simulink model "Color_Space"  (R2013b)
settings: Solver=ode45  StartTime=0.0  StopTime=384*512  RelTol=1e-3
undefined symbols (not defined in the file or in its folder): gray
libraries: xbsIndex_r4 x29, dspsigattribs x9, visionsinks x3, visionsources x1
settings Model: Creator=Sechw  LastModifiedBy=Sechw

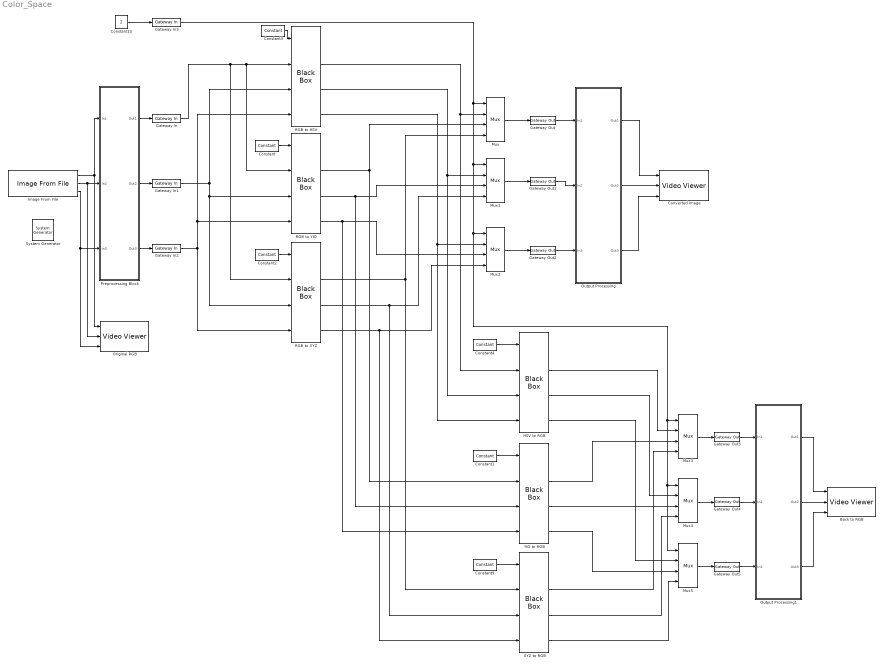
== system Color_Space ==
  " System Generator" : xbsIndex_r4/ System Generator  Tag=genX  xilinxfamily=virtex5  part=xc5vlx110t  speed=-1  package=ff1136  synthesis_tool=XST  clock_wrapper=Clock Enables  directory=./netlist  proj_type=Project Navigator  Synth_file=XST Defaults  Impl_file=ISE Defaults  testbench=off  simulink_period=1  sysclk_period=10  dcm_input_clock_period=10  incr_netlist=off  trim_vbits=Everywhere in SubSystem  dbl_ovrd=According to Block Masks  core_generation=According to Block Masks  run_coregen=off  deprecated_control=off  eval_field=0  block_type=sysgen
  Back to RGB : visionsinks/Video Viewer  inputType=Obsolete7b  imagePorts=Separate color signals  useColorMap=off  colormapValue=gray(256)  specRange=off  minInputVal=0  maxInputVal=255  FigPos=[230 612 675 424]  AxisZoom=on  trueSizedOnce=off  OpenAtMdlStart=on  DefaultConfigurationName=vipscopes.VideoViewerScopeCfg
  Constant{,1..4,9} (6 alike) : xbsIndex_r4/Constant  const=0  gui_display_data_type=Boolean  arith_type=Boolean  n_bits=16  bin_pt=14  preci_type=Single  exp_width=8  frac_width=24  explicit_period=off  period=1  equ=P=C  opselect=C  inp2=PCIN>>17  opr=+  inp1=P  carry=CIN  dbl_ovrd=off  block_type=constant
  Constant13 : Constant  Value=2
  Converted Image : visionsinks/Video Viewer  inputType=Obsolete7b  imagePorts=Separate color signals  useColorMap=off  colormapValue=gray(256)  specRange=off  minInputVal=0  maxInputVal=255  FigPos=[197 708 647 463]  AxisZoom=on  trueSizedOnce=off  OpenAtMdlStart=on  DefaultConfigurationName=vipscopes.VideoViewerScopeCfg
  Gateway In : xbsIndex_r4/Gateway In  gui_display_data_type=Fixed-point  arith_type=Unsigned  n_bits=8  bin_pt=0  preci_type=Double  exp_width=8  frac_width=24  quantization="Round  (unbiased: +/- Inf)"  overflow=Saturate  period=1  dbl_ovrd=off  timing_constraint=None  locs_specified=off  LOCs={}  UseAsADC=off  ADCChannel='1'  inherit_from_input=off  hdl_port=on  block_type=gatewayin
  Gateway In1 : xbsIndex_r4/Gateway In  gui_display_data_type=Fixed-point  arith_type=Unsigned  n_bits=8  bin_pt=0  preci_type=Double  exp_width=8  frac_width=24  quantization="Round  (unbiased: +/- Inf)"  overflow=Saturate  period=1  dbl_ovrd=off  timing_constraint=None  locs_specified=off  LOCs={}  UseAsADC=off  ADCChannel='1'  inherit_from_input=off  hdl_port=on  block_type=gatewayin
  Gateway In2 : xbsIndex_r4/Gateway In  gui_display_data_type=Fixed-point  arith_type=Unsigned  n_bits=8  bin_pt=0  preci_type=Double  exp_width=8  frac_width=24  quantization="Round  (unbiased: +/- Inf)"  overflow=Saturate  period=1  dbl_ovrd=off  timing_constraint=None  locs_specified=off  LOCs={}  UseAsADC=off  ADCChannel='1'  inherit_from_input=off  hdl_port=on  block_type=gatewayin
  Gateway In3 : xbsIndex_r4/Gateway In  gui_display_data_type=Fixed-point  arith_type=Unsigned  n_bits=2  bin_pt=0  preci_type=Single  exp_width=8  frac_width=24  quantization="Round  (unbiased: +/- Inf)"  overflow=Saturate  period=1  dbl_ovrd=off  timing_constraint=None  locs_specified=off  LOCs={}  UseAsADC=off  ADCChannel='1'  inherit_from_input=off  hdl_port=on  block_type=gatewayin
  Gateway Out{,1..5} (6 alike) : xbsIndex_r4/Gateway Out  inherit_from_input=on  hdl_port=on  timing_constraint=None  locs_specified=off  LOCs={}  UseAsDAC=off  DACChannel='1'  block_type=gatewayout
  HSV to RGB : xbsIndex_r4/Black Box  init_code=hsvtorgb_fixpt_xsgbbxcfg  sim_method=ISE Simulator  verbose=off  block_type=blackbox2
  Image From File : visionsources/Image From File  Tag=vipblks_nd  FileName=C:\Users\Sechw\Documents\MATLAB\4440\peppers.png  imagePorts=Separate color signals  Ts=inf  ImageDataType=Inherit from input image  Signed=on  WordLength=16  sdImageDataType=uint(8)  FractionLengthMode=User-defined  FractionLength=15  OutPortLabels=R|G|B
  Mux{,1..5} (6 alike) : xbsIndex_r4/Mux  inputs=3  en=off  latency=0  precision=Full  arith_type=Unsigned  n_bits=16  bin_pt=14  quantization=Truncate  overflow=Wrap  dbl_ovrd=off  block_type=mux
  Original RGB : visionsinks/Video Viewer  inputType=Obsolete7b  imagePorts=Separate color signals  useColorMap=off  colormapValue=gray(256)  specRange=off  minInputVal=0  maxInputVal=255  FigPos=[800 621 504 461]  AxisZoom=on  trueSizedOnce=off  OpenAtMdlStart=on  DefaultConfigurationName=vipscopes.VideoViewerScopeCfg
  Output Processing : Subsystem
  Output Processing1 : Subsystem
  Preprocessing Block : Subsystem
  RGB to HSV : xbsIndex_r4/Black Box  init_code=rgbtohsv_fixpt_xsgbbxcfg  sim_method=ISE Simulator  verbose=off  block_type=blackbox2
  RGB to XYZ : xbsIndex_r4/Black Box  init_code=rgbtoxyz_fixpt_xsgbbxcfg  sim_method=ISE Simulator  verbose=off  block_type=blackbox2
  RGB to YIQ : xbsIndex_r4/Black Box  init_code=rgbtoyiq_fixpt_xsgbbxcfg  sim_method=ISE Simulator  verbose=off  block_type=blackbox2
  XYZ to RGB : xbsIndex_r4/Black Box  init_code=xyztorgb_fixpt_xsgbbxcfg  sim_method=ISE Simulator  verbose=off  block_type=blackbox2
  YIQ to RGB : xbsIndex_r4/Black Box  init_code=yiqtorgb_fixpt_xsgbbxcfg  sim_method=ISE Simulator  verbose=off  block_type=blackbox2
  wires:
  Image From File/1 -> Preprocessing Block/1(In1), Original RGB/1
  Image From File/2 -> Original RGB/2, Preprocessing Block/2(In2)
  Image From File/3 -> Original RGB/3, Preprocessing Block/3(In3)
  Preprocessing Block/1(Out1) -> Gateway In/1
  Preprocessing Block/2(Out2) -> Gateway In1/1
  Preprocessing Block/3(Out3) -> Gateway In2/1
  Gateway Out/1 -> Output Processing/1(In1)
  Gateway Out1/1 -> Output Processing/2(In2)
  Gateway Out2/1 -> Output Processing/3(In3)
  Output Processing/1(Out1) -> Converted Image/1
  Output Processing/2(Out2) -> Converted Image/2
  Output Processing/3(Out3) -> Converted Image/3
  Gateway Out3/1 -> Output Processing1/1(In1)
  Gateway Out4/1 -> Output Processing1/2(In2)
  Gateway Out5/1 -> Output Processing1/3(In3)
  Output Processing1/1(Out1) -> Back to RGB/1
  Output Processing1/2(Out2) -> Back to RGB/2
  Output Processing1/3(Out3) -> Back to RGB/3
  Constant1/1 -> YIQ to RGB/1
  Constant2/1 -> RGB to XYZ/1
  Mux/1 -> Gateway Out/1
  Mux1/1 -> Gateway Out1/1
  Mux2/1 -> Gateway Out2/1
  Constant9/1 -> XYZ to RGB/1
  Mux3/1 -> Gateway Out3/1
  Mux4/1 -> Gateway Out4/1
  Mux5/1 -> Gateway Out5/1
  Constant13/1 -> Gateway In3/1
  Constant3/1 -> RGB to HSV/1
  Constant4/1 -> HSV to RGB/1
  Gateway In/1 -> RGB to YIQ/2, RGB to HSV/2, RGB to XYZ/2
  Constant/1 -> RGB to YIQ/1
  Gateway In1/1 -> RGB to HSV/3, RGB to XYZ/3, RGB to YIQ/3
  Gateway In2/1 -> RGB to YIQ/4, RGB to HSV/4, RGB to XYZ/4
  RGB to HSV/2 -> HSV to RGB/2, Mux/2
  RGB to HSV/3 -> HSV to RGB/3, Mux1/2
  RGB to HSV/4 -> HSV to RGB/4, Mux2/2
  RGB to YIQ/2 -> Mux/3, YIQ to RGB/2
  RGB to YIQ/3 -> YIQ to RGB/3, Mux1/3
  RGB to YIQ/4 -> YIQ to RGB/4, Mux2/3
  RGB to XYZ/2 -> XYZ to RGB/2, Mux/4
  RGB to XYZ/3 -> XYZ to RGB/3, Mux1/4
  RGB to XYZ/4 -> XYZ to RGB/4, Mux2/4
  Gateway In3/1 -> Mux5/1, Mux4/1, Mux3/1, Mux2/1, Mux1/1, Mux/1
  HSV to RGB/2 -> Mux3/2
  HSV to RGB/3 -> Mux4/2
  HSV to RGB/4 -> Mux5/2
  YIQ to RGB/2 -> Mux3/3
  YIQ to RGB/3 -> Mux4/3
  YIQ to RGB/4 -> Mux5/3
  XYZ to RGB/2 -> Mux3/4
  XYZ to RGB/3 -> Mux4/4
  XYZ to RGB/4 -> Mux5/4

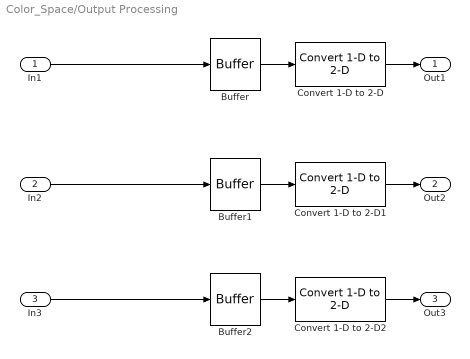
== system Color_Space/Output Processing ==
  In1 : Inport
  In2 : Inport  Port=2
  In3 : Inport  Port=3
  Buffer : Buffer  N=384*512  TreatMby1Signals=One channel
  Buffer1 : Buffer  N=384*512  TreatMby1Signals=One channel
  Buffer2 : Buffer  N=384*512  TreatMby1Signals=One channel
  Convert 1-D to 2-D : dspsigattribs/Convert 1-D to 2-D  M=384  N=512  frameBasedOut=off
  Convert 1-D to 2-D1 : dspsigattribs/Convert 1-D to 2-D  M=384  N=512  frameBasedOut=off
  Convert 1-D to 2-D2 : dspsigattribs/Convert 1-D to 2-D  M=384  N=512  frameBasedOut=off
  Out1 : Outport
  Out2 : Outport  Port=2
  Out3 : Outport  Port=3
  wires:
  Convert 1-D to 2-D2/1 -> Out3/1
  Convert 1-D to 2-D1/1 -> Out2/1
  Buffer1/1 -> Convert 1-D to 2-D1/1
  Buffer2/1 -> Convert 1-D to 2-D2/1
  Buffer/1 -> Convert 1-D to 2-D/1
  Convert 1-D to 2-D/1 -> Out1/1
  In1/1 -> Buffer/1
  In2/1 -> Buffer1/1
  In3/1 -> Buffer2/1

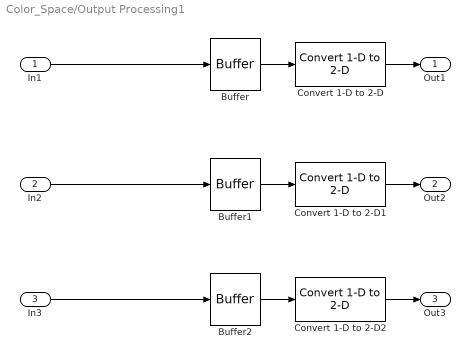
== system Color_Space/Output Processing1 ==
  In1 : Inport
  In2 : Inport  Port=2
  In3 : Inport  Port=3
  Buffer : Buffer  N=384*512  TreatMby1Signals=One channel
  Buffer1 : Buffer  N=384*512  TreatMby1Signals=One channel
  Buffer2 : Buffer  N=384*512  TreatMby1Signals=One channel
  Convert 1-D to 2-D : dspsigattribs/Convert 1-D to 2-D  M=384  N=512  frameBasedOut=off
  Convert 1-D to 2-D1 : dspsigattribs/Convert 1-D to 2-D  M=384  N=512  frameBasedOut=off
  Convert 1-D to 2-D2 : dspsigattribs/Convert 1-D to 2-D  M=384  N=512  frameBasedOut=off
  Out1 : Outport
  Out2 : Outport  Port=2
  Out3 : Outport  Port=3
  wires:
  Convert 1-D to 2-D2/1 -> Out3/1
  Convert 1-D to 2-D1/1 -> Out2/1
  Buffer1/1 -> Convert 1-D to 2-D1/1
  Buffer2/1 -> Convert 1-D to 2-D2/1
  Buffer/1 -> Convert 1-D to 2-D/1
  Convert 1-D to 2-D/1 -> Out1/1
  In1/1 -> Buffer/1
  In2/1 -> Buffer1/1
  In3/1 -> Buffer2/1

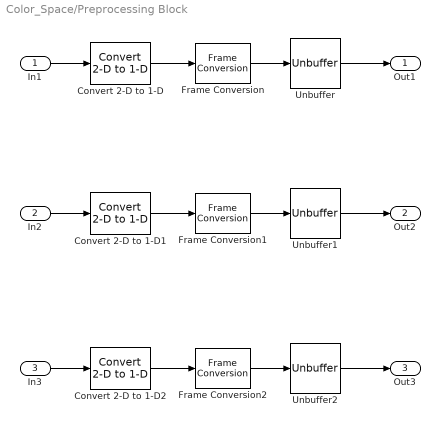
== system Color_Space/Preprocessing Block ==
  In1 : Inport
  In2 : Inport  Port=2
  In3 : Inport  Port=3
  Convert 2-D to 1-D : dspsigattribs/Convert 2-D to 1-D
  Convert 2-D to 1-D1 : dspsigattribs/Convert 2-D to 1-D
  Convert 2-D to 1-D2 : dspsigattribs/Convert 2-D to 1-D
  Frame Conversion : FrameConversion
  Frame Conversion1 : FrameConversion
  Frame Conversion2 : FrameConversion
  Unbuffer : Unbuffer  SampleBasedProcessing=Same as frame based
  Unbuffer1 : Unbuffer  SampleBasedProcessing=Same as frame based
  Unbuffer2 : Unbuffer  SampleBasedProcessing=Same as frame based
  Out1 : Outport
  Out2 : Outport  Port=2
  Out3 : Outport  Port=3
  wires:
  In1/1 -> Convert 2-D to 1-D/1
  Frame Conversion1/1 -> Unbuffer1/1
  Convert 2-D to 1-D1/1 -> Frame Conversion1/1
  In2/1 -> Convert 2-D to 1-D1/1
  Unbuffer1/1 -> Out2/1
  Frame Conversion2/1 -> Unbuffer2/1
  In3/1 -> Convert 2-D to 1-D2/1
  Convert 2-D to 1-D2/1 -> Frame Conversion2/1
  Unbuffer2/1 -> Out3/1
  Unbuffer/1 -> Out1/1
  Frame Conversion/1 -> Unbuffer/1
  Convert 2-D to 1-D/1 -> Frame Conversion/1
